simulink model "simu_AtoB"  (R2023a)
settings: Solver=FixedStepAuto  StartTime=0.0  StopTime=10  FixedStep=1e-3  RelTol=1e-3
undefined symbols (not defined in the file): Kalpha, Kbeta, Krho, longueur, theta_a, thetastar, x_a, xstar, y_a, ystar
settings Model: Creator=daneydem1u  LastModifiedBy=daneydem1u

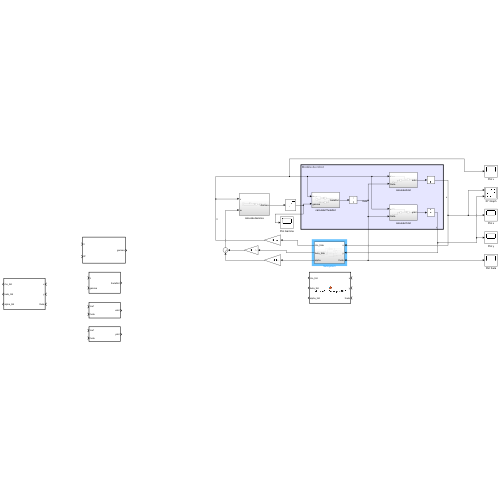
[thumbnail: Simulink's stored preview of the top-level diagram]
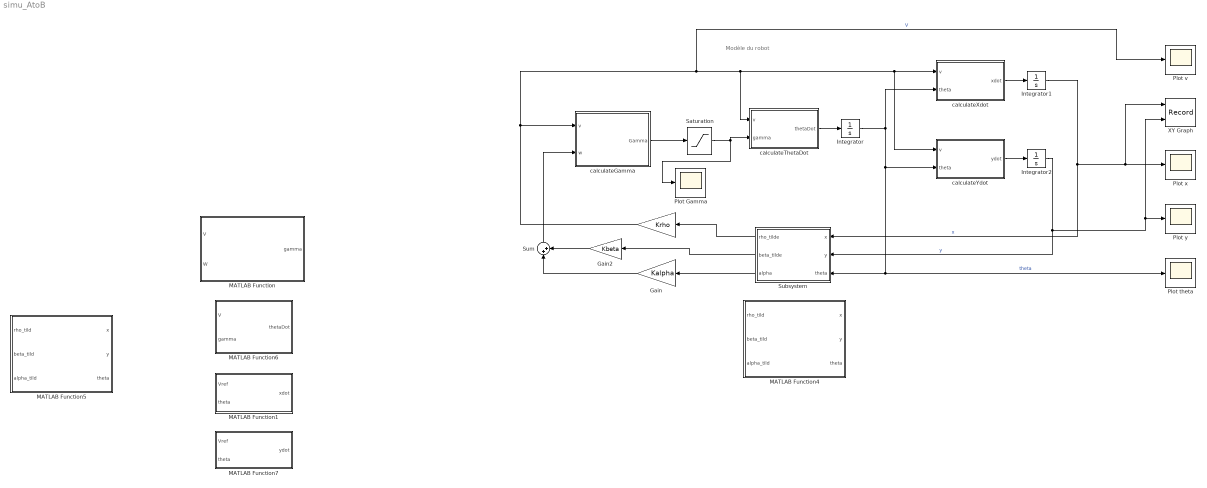
== system simu_AtoB ==
  note: Modèle du robot
  " " : Gain  Gain=Krho
  Gain : Gain  Gain=Kalpha
  Gain2 : Gain  Gain=Kbeta
  Integrator : Integrator  InitialCondition=theta_a
  Integrator1 : Integrator  InitialCondition=x_a
  Integrator2 : Integrator  InitialCondition=y_a
  MATLAB Function : MATLAB Function  TreatAsAtomicUnit=on
  MATLAB Function1 : MATLAB Function  TreatAsAtomicUnit=on
  MATLAB Function4 : MATLAB Function  TreatAsAtomicUnit=on
  MATLAB Function5 : MATLAB Function  TreatAsAtomicUnit=on
  MATLAB Function6 : MATLAB Function  TreatAsAtomicUnit=on
  MATLAB Function7 : MATLAB Function  TreatAsAtomicUnit=on
  Plot Gamma : Scope
  Plot theta : Scope
  Plot v : Scope
  Plot x : Scope
  Plot y : Scope
  Saturation : Saturate  UpperLimit=pi/4  LowerLimit=-pi/4
  Subsystem : Subsystem
  Sum : Sum  Inputs=|++
  XY Graph : Record  FileSettingsInternal="{\"entries\":[{\"content\":{\"excelSettings\":{\"content\":{},\"type\":\"Streamout.ExcelSettings\"}},\"type\":\"Streamout.FileSettingStorage\",\"uuid\":\"3953bc1f-c420-42c2-a4d0-df2908d07df4\"}],\"packageUris\":[\"http://schema.mathworks.com/mf0/streamout_blocks/R2020a\"],\"version\":\"1.0\"}"  Layout=[1 1]  SignalsInternal="{\"entries\":[{\"content\":{\"signals\":[{\"content\":{\"blockPath\":[\"simu_AtoB/XY Graph\"],\"dimensions\":[1],\"domain\":\"simu_AtoB/XY Graph\",\"lineColor\":\"#a2142f\",\"plots\":[1],\"port\":1,\"sid\":[\"\"],\"signalID\":5722,\"signalName\":\"x\"},\"type\":\"RecordBlkView.Signal\",\"uuid\":\"1931e263-2d32-4d49-8891-a7855915e3d7\"},{\"content\":{\"blockPath\":[\"simu_AtoB/XY Graph\"],\"dimensions\":[1],\"domain\":\"simu_AtoB/XY Graph\",\"lineColor\":\"#139fff\",\"plots\":[1],\"port\":2,\"sid\":[\"\"],\"signalID\":5726,\"signalName\":\"y\"},\"type\":\"RecordBlkView.Signal\",\"uuid\":\"24751e08-3c34-4a57-89dd-e8ca9477e8d6\"}]},\"type\":\"RecordBlkView.InputSignals\",\"uuid\":\"d09ba45a-57a1-4630-9d3a-53c37102ddb1\"}],\"packageUris\":[\"http://schema.mathworks.com/mf0/streamout_blocks/R2020a\"],\"version\":\"1.0\"}"  VisualizationBindings="{\"xyplotplugin\":{\"info\":[{\"series\":[{\"bindingParametersList\":[{\"parameter\":\"X-Axis\",\"signalID\":5722,\"signalName\":\"x\"},{\"parameter\":\"Y-Axis\",\"signalID\":5726,\"signalName\":\"y\"}],\"seriesID\":19815}],\"subplotID\":1}]}}"  CompatibilityTag=XY
  calculateGamma : Subsystem
  calculateThetaDot : Subsystem
  calculateXdot : Subsystem
  calculateYdot : Subsystem
  wires:
  " "/1 -> calculateGamma/1(v), Plot v/1, calculateThetaDot/1(v), calculateYdot/1(v), calculateXdot/1(v)  "V"
  Integrator/1 -> Subsystem/3(theta), Plot theta/1, calculateYdot/2(theta), calculateXdot/2(theta)  "theta"
  calculateXdot/1(xdot) -> Integrator1/1
  calculateYdot/1(ydot) -> Integrator2/1
  Integrator1/1 -> Subsystem/1(x), XY Graph/1, Plot x/1  "x"
  Integrator2/1 -> Subsystem/2(y), XY Graph/2, Plot y/1  "y"
  Gain2/1 -> Sum/2
  Gain/1 -> Sum/1
  Saturation/1 -> Plot Gamma/1, calculateThetaDot/2(gamma)
  calculateGamma/1(Gamma) -> Saturation/1
  Sum/1 -> calculateGamma/2(w)
  calculateThetaDot/1(thetaDot) -> Integrator/1
  Subsystem/3(alpha) -> Gain/1
  Subsystem/2(beta_tilde) -> Gain2/1
  Subsystem/1(rho_tilde) -> " "/1

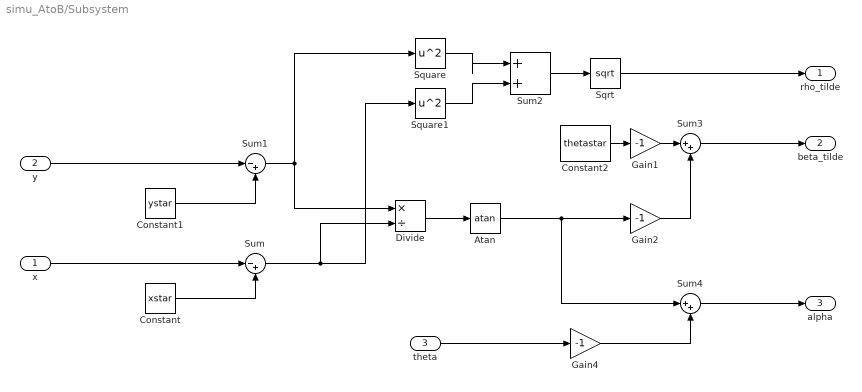
== system simu_AtoB/Subsystem ==
  x : Inport
  y : Inport  Port=2
  theta : Inport  Port=3
  Atan : Trigonometry  Operator=atan
  Constant : Constant  Value=xstar
  Constant1 : Constant  Value=ystar
  Constant2 : Constant  Value=thetastar
  Divide : Product  Inputs=*/
  Gain1 : Gain  Gain=-1
  Gain2 : Gain  Gain=-1
  Gain4 : Gain  Gain=-1
  Sqrt : Sqrt
  Square : Math  Operator=square
  Square1 : Math  Operator=square
  Sum : Sum  Inputs=|-+
  Sum1 : Sum  Inputs=|-+
  Sum2 : Sum  Inputs=|++
  Sum3 : Sum  Inputs=|++
  Sum4 : Sum  Inputs=|++
  rho_tilde : Outport
  beta_tilde : Outport  Port=2
  alpha : Outport  Port=3
  wires:
  Sqrt/1 -> rho_tilde/1
  Square/1 -> Sum2/1
  Sum/1 -> Divide/2, Square1/1
  Constant/1 -> Sum/2
  x/1 -> Sum/1
  Constant1/1 -> Sum1/2
  Square1/1 -> Sum2/2
  y/1 -> Sum1/1
  Sum1/1 -> Divide/1, Square/1
  Sum2/1 -> Sqrt/1
  theta/1 -> Gain4/1
  Constant2/1 -> Gain1/1
  Divide/1 -> Atan/1
  Gain4/1 -> Sum4/2
  Sum3/1 -> beta_tilde/1
  Sum4/1 -> alpha/1
  Gain1/1 -> Sum3/1
  Atan/1 -> Gain2/1, Sum4/1
  Gain2/1 -> Sum3/2

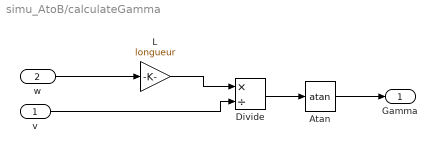
== system simu_AtoB/calculateGamma ==
  v : Inport
  w : Inport  Port=2
  Atan : Trigonometry  Operator=atan
  Divide : Product  Inputs=*/
  L : Gain  Gain=longueur
  Gamma : Outport
  wires:
  Divide/1 -> Atan/1
  v/1 -> Divide/2
  Atan/1 -> Gamma/1
  L/1 -> Divide/1
  w/1 -> L/1

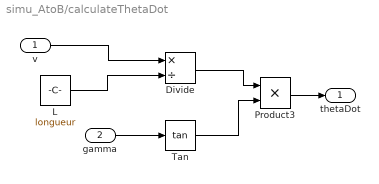
== system simu_AtoB/calculateThetaDot ==
  v : Inport
  gamma : Inport  Port=2
  Divide : Product  Inputs=*/
  L : Constant  Value=longueur
  Product3 : Product
  Tan : Trigonometry  Operator=tan
  thetaDot : Outport
  wires:
  Tan/1 -> Product3/2
  Divide/1 -> Product3/1
  gamma/1 -> Tan/1
  L/1 -> Divide/2
  Product3/1 -> thetaDot/1
  v/1 -> Divide/1

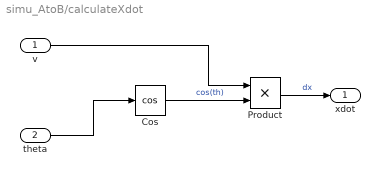
== system simu_AtoB/calculateXdot ==
  v : Inport
  theta : Inport  Port=2
  Cos : Trigonometry  Operator=cos
  Product : Product
  xdot : Outport
  wires:
  v/1 -> Product/1
  theta/1 -> Cos/1
  Cos/1 -> Product/2  "cos(th)"
  Product/1 -> xdot/1  "dx"

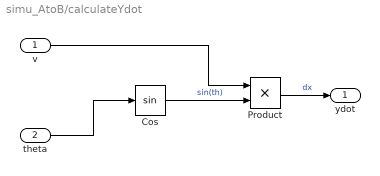
== system simu_AtoB/calculateYdot ==
  v : Inport
  theta : Inport  Port=2
  Cos : Trigonometry
  Product : Product
  ydot : Outport
  wires:
  v/1 -> Product/1
  theta/1 -> Cos/1
  Cos/1 -> Product/2  "sin(th)"
  Product/1 -> ydot/1  "dx"

== matlab function simu_AtoB/MATLAB Function1 ==
  data: Vref input; xdot output; theta input
function xdot = calculateXdot(Vref, theta)
    xdot = Vref * cos(theta);
end

== matlab function simu_AtoB/MATLAB Function ==
  data: V input; gamma output; W input; longueur parameter
function gamma = calculateGamma(V, W, longueur)
    gamma = atan((W * longueur) / V);
end

== matlab function simu_AtoB/MATLAB Function4 ==
  data: x input; rho_tild output; y input; theta input; beta_tild output; alpha_tild output; xstar parameter; ystar parameter; thetastar parameter
function [rho_tild, beta_tild, alpha_tild] = calculateRhoBetaAlphaTILD(x, y, theta, xstar, ystar, thetastar)
    dx = xstar - x;
    dy = ystar - y;

    rho_tild = sqrt(dx^2 + dy^2);
    angle_to_target = atan2(dy, dx);

    alpha_tild = angle_to_target - theta;
    beta_tild = - thetastar - angle_to_target;

end

== matlab function simu_AtoB/MATLAB Function5 ==
  data: x input; rho_tild output; y input; theta input; beta_tild output; alpha_tild output; xstar parameter; ystar parameter; thetastar parameter
function [rho_tild, beta_tild, alpha_tild] = calculateRhoBetaAlphaTILD(x, y, theta, xstar, ystar, thetastar)
    dx = xstar - x;
    dy = ystar - y;

    rho_tild = sqrt(dx^2 + dy^2);
    beta_tild = -atan(dy/dx) - thetastar;
    alpha_tild = atan(dy/dx) - theta;
end

== matlab function simu_AtoB/MATLAB Function6 ==
  data: V input; thetaDot output; gamma input; longueur parameter
function thetaDot = calculateThetaDot(V, gamma, longueur)
    % Calcul de thetaDot
    thetaDot = V * tan(gamma) / longueur;
end

== matlab function simu_AtoB/MATLAB Function7 ==
  data: Vref input; ydot output; theta input
function ydot = calculateYdot(Vref, theta)
    ydot = Vref * sin(theta);
end
